simulink model "ConsignaSuavizada"  (R2023b)
settings: Solver=VariableStepAuto  StartTime=0.0  StopTime=16  MaxStep=1e-5  RelTol=1e-3
settings Model: Creator=Home  LastModifiedBy=Home

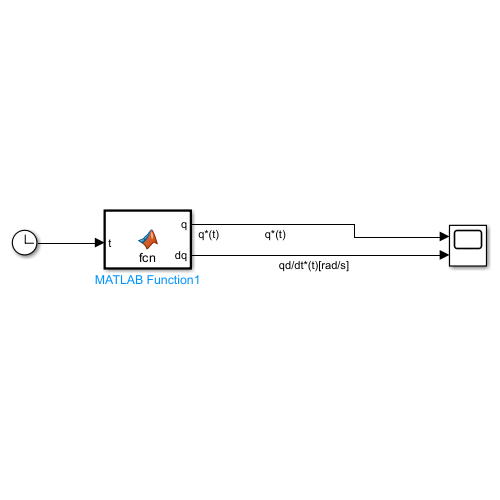
[thumbnail: Simulink's stored preview of the top-level diagram]
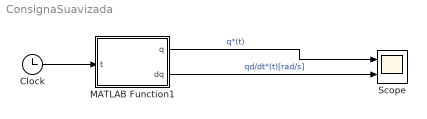
== system ConsignaSuavizada ==
  Clock : Clock
  MATLAB Function1 : MATLAB Function  TreatAsAtomicUnit=on
  Scope : Scope  NumInputPorts=2
  wires:
  Clock/1 -> MATLAB Function1/1(t)
  MATLAB Function1/1(q) -> Scope/1  "q*(t)"
  MATLAB Function1/2(dq) -> Scope/2  "qd/dt*(t)[rad/s]"

== matlab function ConsignaSuavizada/MATLAB Function1 ==
  data: t input; q output; dq output
function [q, dq] = fcn(t)
    % Salidas:
    % q  -> Consigna de posición [rad]
    % dq -> Consigna de velocidad [rad/s]
    
    % Constantes
    max_pos = 2 * pi;       % Posición máxima [rad]
    ramp_time = 0.1;       % Tiempo de rampa [s]
    plateau_time = 5;       % Duración de velocidad constante [s]
    total_time = 2 * plateau_time + 2 * ramp_time; % Tiempo total [s]
    
    % Velocidad máxima
    max_vel = max_pos / plateau_time; % Velocidad constante [rad/s]
    
    % Inicialización de variables de salida
    dq = 0; % Velocidad
    q = 0;  % Posición
    
    % Lógica de perfil de velocidad
    if t < ramp_time
        % Rampa de aceleración (inicio de movimiento)
        dq = max_vel * (t / ramp_time);
    elseif t >= ramp_time && t < plateau_time + ramp_time
        % Velocidad constante positiva (incremento lineal de posición)
        dq = max_vel;
    elseif t >= plateau_time + ramp_time && t < plateau_time + 2 * ramp_time
        % Rampa de desaceleración positiva (fin del incremento)
        dq = max_vel * (1 - (t - plateau_time - ramp_time) / ramp_time);
    elseif t >= plateau_time + 2 * ramp_time && t < 2 * plateau_time + 2 * ramp_time
        % Velocidad cero (mantener posición constante en 2*pi)
        dq = 0;
    elseif t >= 2 * plateau_time + 2 * ramp_time && t < 2 * plateau_time + 3 * ramp_time
        % Rampa de aceleración negativa (inicio del decremento)
        dq = -max_vel * ((t - 2 * plateau_time - 2 * ramp_time) / ramp_time);
    elseif t >= 2 * plateau_time + 3 * ramp_time && t < 3 * plateau_time + 3 * ramp_time
        % Velocidad constante negativa (decremento lineal de posición)
        dq = -max_vel;
    elseif t >= 3 * plateau_time + 3 * ramp_time && t < 3 * plateau_time + 4 * ramp_time
        % Rampa de desaceleración negativa (fin del decremento)
        dq = -max_vel * (1 - (t - 3 * plateau_time - 3 * ramp_time) / ramp_time);
    else
        % Fuera del rango definido, posición constante en 0
        dq = 0;
    end
    
    % Integración de la velocidad para obtener la posición
    % Usamos persistencia para mantener los valores previos
    persistent q_prev t_prev;
    if isempty(q_prev) || isempty(t_prev)
        q_prev = 0;
        t_prev = 0;
    end
    
    dt = t - t_prev; % Paso de tiempo
    if dt > 0
        q = q_prev + dq * dt; % Integración discreta
    else
        q = q_prev;
    end
    
    % Actualizar valores previos
    q_prev = q;
    t_prev = t;
end
